simulink model "sampling"  (R2014b)
settings: Solver=ode3  StartTime=0.0  StopTime=sim_time  RelTol=1e-3
values from neighbouring files (symbols this model uses):
  A = input('Enter max amplitude of signal = ')    [mfile_sampling.m]
  F = input('Enter the sampling frequency = ')    [mfile_sampling.m]
  f = input('Enter the frequency of signal = ')    [mfile_sampling.m]    (also in sampling_demo.m = 50)
  fc = input('Enter the lowpass filter cutoff frequency = ')    [mfile_sampling.m]
  I = 2*A/(L-1)    [mfile_sampling.m]
  L = 2^qbits    [mfile_sampling.m]
libraries: dspxfrm3 x3, dspquant2 x2, dsparch4 x1, simulink x1
settings Model: Creator=Mukhtar Hussain  LastModifiedBy=Mukhtar Hussain

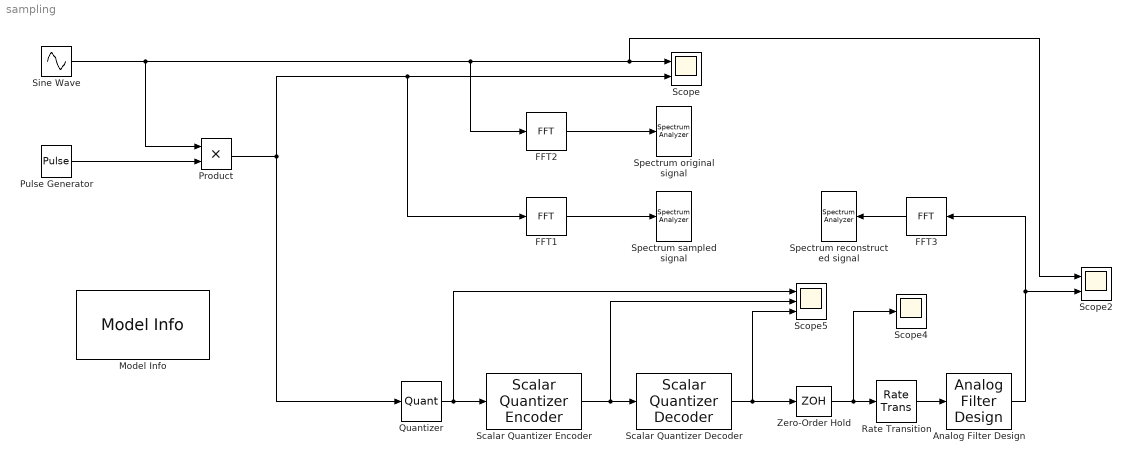
== system sampling ==
  Analog Filter Design : dsparch4/Analog Filter Design  method=Butterworth  filttype=Lowpass  N=8  Wlo=2*pi*fc  Whi=80  Rp=2  Rs=40
  FFT1 : dspxfrm3/FFT  CompMethod=Table lookup  TableOpt=NEW  TableOptActive=Speed  BitRevOrder=off  InheritFFTLength=on  FFTLength=512  WrapInput=on  RowConvenienceOn=on  FFTImplementation=Auto  SkipNorm=on  firstCoeffDataTypeStr=Inherit: Same word length as input  firstCoeffLastDataTypeStr=Inherit: Same word length as input  outputMin=[]  outputMax=[]  roundingMode=Floor  overflowMode=off
  FFT2 : dspxfrm3/FFT  CompMethod=Table lookup  TableOpt=NEW  TableOptActive=Speed  BitRevOrder=off  InheritFFTLength=on  FFTLength=512  WrapInput=on  RowConvenienceOn=on  FFTImplementation=Auto  SkipNorm=off  firstCoeffDataTypeStr=Inherit: Same word length as input  firstCoeffLastDataTypeStr=Inherit: Same word length as input  outputMin=[]  outputMax=[]  roundingMode=Floor  overflowMode=off
  FFT3 : dspxfrm3/FFT  CompMethod=Table lookup  TableOpt=NEW  TableOptActive=Speed  BitRevOrder=off  InheritFFTLength=on  FFTLength=512  WrapInput=on  RowConvenienceOn=on  FFTImplementation=Auto  SkipNorm=off  firstCoeffDataTypeStr=Inherit: Same word length as input  firstCoeffLastDataTypeStr=Inherit: Same word length as input  outputMin=[]  outputMax=[]  roundingMode=Floor  overflowMode=off
  Model Info : simulink/Model-Wide Utilities/Model Info  Frame=on  DisplayStringWithTags=|  HorizontalTextAlignment=Center  LeftAlignmentValue=0.5  SourceBlockDiagram=sampling  TagMaxNumber=20
      | Sampling & 
      | Reconstruction
      | by
      | %<Creator>
  Product : Product
  Pulse Generator : DiscretePulseGenerator  PulseType=Time based  Period=1/F  PulseWidth=10
  Quantizer : Quantizer  QuantizationInterval=2*A/L  LinearizeAsGain=off
  Rate Transition : RateTransition  OutPortSampleTimeOpt=Inherit
  Scalar Quantizer Decoder : dspquant2/Scalar Quantizer Decoder  invalidin=Clip  CBsource=Specify via dialog  codebook=[-A:I:A]  dataType=double  isSigned=on  wordLen=16  udDataType=sfix(16)  fracBitsMode=Best precision  numFracBits=11  OutDataTypeStr=double  LastOutDataTypeStr=double
  Scalar Quantizer Encoder : dspquant2/Scalar Quantizer Encoder  paramSrc=Specify via dialog  partType=Unbounded  BBoundary=[-5:10/15:5]  UBoundary=[-A:I:A]  SearchMethod=Binary  tieBreakRule=Choose the lower index  outQU=off  outQError=off  codebook=[-5:10/16:5]  outStatus=off  invalidin=Clip  idtype=uint32  roundingMode=Floor  overflowMode=off
  Scope : Scope  NumInputPorts=2
      settings: ShowLegends=on  YMin=-5~-5  YMax=5~5
  Scope2 : Scope  NumInputPorts=2
      settings: ShowLegends=on  YMin=-5~-5  YMax=5~5  SaveName=ScopeData2
  Scope4 : Scope
      settings: ShowLegends=on  SaveName=ScopeData4
  Scope5 : Scope  NumInputPorts=3
      settings: ShowLegends=on  YMin=-5~-5~-5  YMax=5~5~5  SaveName=ScopeData5
  Sine Wave : Sin  Amplitude=A  Frequency=2*pi*f  Phase=pi/2  SampleTime=0
  Spectrum original signal : SpectrumAnalyzer
  Spectrum reconstructed signal : SpectrumAnalyzer
  Spectrum sampled signal : SpectrumAnalyzer
  Zero-Order Hold : ZeroOrderHold  SampleTime=1/F
  wires:
  Pulse Generator/1 -> Product/2
  Quantizer/1 -> Scope5/1, Scalar Quantizer Encoder/1
  FFT2/1 -> Spectrum original signal/1
  Product/1 -> Quantizer/1, Scope/2, FFT1/1
  Scalar Quantizer Decoder/1 -> Scope5/3, Zero-Order Hold/1
  Zero-Order Hold/1 -> Scope4/1, Rate Transition/1
  Scalar Quantizer Encoder/1 -> Scope5/2, Scalar Quantizer Decoder/1
  Rate Transition/1 -> Analog Filter Design/1
  Analog Filter Design/1 -> FFT3/1, Scope2/2
  FFT3/1 -> Spectrum reconstructed signal/1
  FFT1/1 -> Spectrum sampled signal/1
  Sine Wave/1 -> Product/1, Scope2/1, Scope/1, FFT2/1
